simulink model "flightControlSystem"  (R2023b)
settings: Solver=ode3  StartTime=0  StopTime=TFinal  FixedStep=Ts  RelTol=1e-3  EnableMultiTasking=on
undefined symbols (not defined in the file): codertarget, Controller, DiscIntNeverNeededParam, Discrete, Estimator, g, gray, init, Sensors, strel, Time, Ts, var_acc_angle_N, var_bias_gyr_N, var_gyro_p_N, Vehicle
libraries: simulink x38, slpidlib x5, ctrlSharedLib x4, sharedtransform x3, simulink_extras x1, visionmorphops x1, parrotlib x1
(part 3 of 3)

== matlab function flightControlSystem/Control System/Path Planning/Drone Course Control/Z_COMMAND ==
  data: TARGET_DETECT input; Z_estimate input; TAKE_OFF_DRONE_PREVIOUSLY input; Z_command output; TAKE_OFF_PRECHECK_STATUS output
function [Z_command, TAKE_OFF_PRECHECK_STATUS]  = Y_command_function(TARGET_DETECT, Z_estimate, TAKE_OFF_DRONE_PREVIOUSLY)

    % Variable declaration
    persistent TAKE_OFF_PRECHECK;
    
    % Initialize TAKE_OFF_PRECHECK if it's not initialized yet
    if isempty(TAKE_OFF_PRECHECK)
        TAKE_OFF_PRECHECK = double(false); % Initialized to False
    end
    
%--------------------------------------------------------------------------
    % Compute Z_command based on conditions
    Z_command = Z_estimate; % Initialized to Z_estimate
    TAKE_OFF_PRECHECK_STATUS = double(false);
%--------------------------------------------------------------------------

    if ~TAKE_OFF_DRONE_PREVIOUSLY
        TAKE_OFF_PRECHECK = double(true);
        
        Z_command = -1.1;
    
    elseif Z_estimate < -0.1 && TARGET_DETECT
        Z_command = Z_command + 0.001;
    
    end

    TAKE_OFF_PRECHECK_STATUS = TAKE_OFF_PRECHECK;

end

== matlab function flightControlSystem/Control System/Path Planning/Centroid_error ==
  data: dist_X_image input; error_x output; X_estimate input; centroid_X_meters output; dist_Y_image input; Y_estimate input; error_y output; centroid_Y_meters output
function [error_x, centroid_X_meters, error_y, centroid_Y_meters]  = Centroid_error(dist_X_image, X_estimate, dist_Y_image, Y_estimate)

error_x = 0.0;
error_y = 0.0;
% Camera image resolution
image_width_pixels = 160;
image_height_pixels = 120;

% Convert centroid X-coordinate to meters
image_width_meters = 1;  % Assuming 1 meter width
pixels_to_meters = image_width_meters / image_width_pixels;
centroid_X_meters = dist_X_image * pixels_to_meters;

% Calculate error in X-coordinate
error_x = centroid_X_meters - X_estimate;


% Convert centroid X-coordinate to meters
image_width_meters = 1;  % Assuming 1 meter width
Y_pixels_to_meters = image_width_meters / image_height_pixels;
centroid_Y_meters = dist_Y_image * Y_pixels_to_meters;

% Calculate error in X-coordinate
error_y = centroid_Y_meters - Y_estimate;

end
